simulink model "accel_sim"  (R2026a)
settings: Solver=ode45  StopTime=15  MaxStep=0.005
PostLoadFcn:
  | p=fileparts(get_param('accel_sim','FileName')); if ~isempty(p), addpath(p, fullfile(p,'lib')); end; if ~exist('G_ratio','var'), assignin('base','G_ratio',4.61); end
InitFcn:
  | if ~exist('G_ratio','var'), assignin('base','G_ratio',4.61); end
StopFcn:
  | if ~exist('SWEEP_MODE','var'),  fprintf('\naccel_sim: 0-75 m at %.2f:1 = %.2f s   (double-click the Scope for the curves)\n',          G_ratio, get_param('accel_sim','SimulationTime'));end
undefined symbols (not defined in the file or in its folder): G_ratio
libraries: simulink x1
settings Model: Creator=Aboud  LastModifiedBy=Aboud

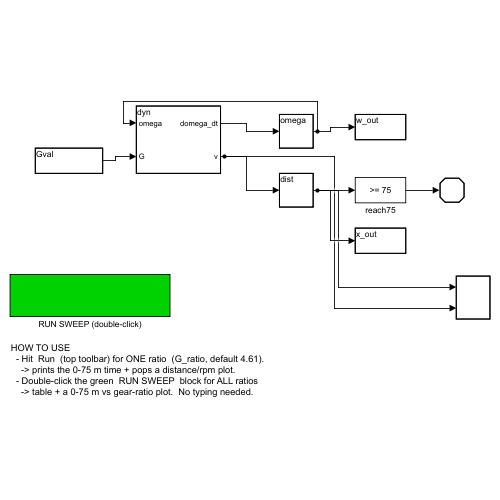
[thumbnail: Simulink's stored preview of the top-level diagram]
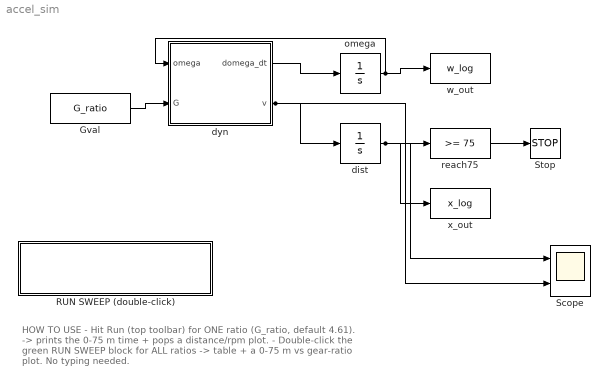
== system accel_sim ==
  note: HOW TO USE
      |   - Hit  Run  (top toolbar) for ONE ratio  (G_ratio, default 4.61).
      |     -> prints the 0-75 m time + pops a distance/rpm plot.
      |   - Double-click the green  RUN SWEEP  block for ALL ratios
      |     -> table + a 0-75 m vs gear-ratio plot.  No typing needed.
  Gval : Constant  Value=G_ratio
  RUN SWEEP (double-click) : Subsystem
      settings: OpenFcn=sweep_accel_sim
  Scope : Scope  NumInputPorts=2
  Stop : Stop
  dist : Integrator
  dyn : MATLAB Function  TreatAsAtomicUnit=on
  omega : Integrator
  reach75 : simulink/Logic and Bit Operations/Compare To Constant  relop=>=  const=75  OutDataTypeStr=boolean
  w_out : ToWorkspace  VariableName=w_log  SaveFormat=Timeseries  SampleTime=-1
  x_out : ToWorkspace  VariableName=x_log  SaveFormat=Timeseries  SampleTime=-1
  wires:
  Gval/1 -> dyn/2(G)
  dyn/1(domega_dt) -> omega/1
  omega/1 -> dyn/1(omega), w_out/1
  dyn/2(v) -> dist/1, Scope/2
  dist/1 -> reach75/1, x_out/1, Scope/1
  reach75/1 -> Stop/1

== system accel_sim/RUN SWEEP (double-click) ==

== matlab function accel_sim/dyn ==
  data: omega input; domega_dt output; G input; v output
function [domega_dt, v] = dyn(omega, G)
%#codegen
r=0.2286; eta=0.794; m=294; rho=1.225; CdA=0.933062; ClA=1.49881; Crr=0.015;
rs=0.483; ra=0.564; hcg=0.3134; L=1.543; g=9.81; redline=6000; Tcap=140; TF=1.5;
Irot=0.0256; Idl=0.0005; Iwh=0.105352; nw=4;
Prpm=[0 1000 2000 3000 4000 5000 6000 ]; Pkw=[0 24 40 50 56 62 68 ];
PDX1=2.1; PDX2=-0.40981; FNOM=667; LMUX=0.65;
n = 1/G;
Iden = Irot + Idl + nw*Iwh*n^2 + m*n^2*r^2;
b = 0.5*rho*r^2*n^2*(CdA + Crr*ClA);
Cc = m*g*Crr;
v = r*n*omega;
rpm = omega*60/(2*pi);
if rpm < 50
    Tm = Tcap;
else
    Pk = interp1(Prpm, Pkw, min(rpm,redline), 'linear', 'extrap');
    Tm = min(Tcap, Pk*9549/rpm);
end
Tm = Tm*eta;
Fdown = 0.5*rho*ClA*v^2;
a = 0; domega_dt = 0;
for it = 1:3
    Fzr = m*g*rs + m*a*hcg/L + Fdown*ra;
    dfz = (Fzr/2 - FNOM)/FNOM;
    mu = max(LMUX*(PDX1 + PDX2*dfz), 0.5);
    Tuse = min(Tm, mu*Fzr*r*n/eta);
    domega_dt = (Tuse - n*r*(b*omega^2 + Cc) - TF)/Iden;
    a = r*n*domega_dt;
end
